simulink model "PD_controller_unit_test"  (R2018b)
settings: Solver=FixedStepAuto  StartTime=0.0  StopTime=100  FixedStep=simParams.sample_time_s  RelTol=1e-3
undefined symbols (not defined in the file): simParams
libraries: PD_Controller_Lib x1, control_command_generation_lib x1, satelliteDynamics_lib x1
settings Model: Creator=colem  LastModifiedBy=colem

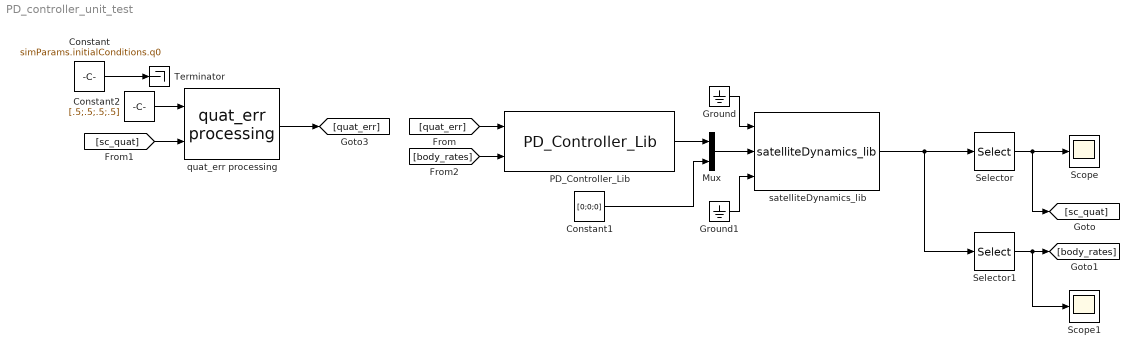
== system PD_controller_unit_test ==
  Constant : Constant  Value=simParams.initialConditions.q0
  Constant1 : Constant  Value=[0;0;0]
  Constant2 : Constant  Value=[.5;.5;.5;.5]
  Ground : Ground
  Ground1 : Ground
  Mux : Mux  Inputs=[3 3]
  PD_Controller_Lib : PD_Controller_Lib/PD_Controller_Lib  SystemSampleTime=-1
  Scope : Scope
  Scope1 : Scope
  Selector : Selector  InputPortWidth=13  IndexOptions=Index vector (dialog)  Indices=[7 8 9 10]  OutputSizes=1
  Selector1 : Selector  InputPortWidth=13  IndexOptions=Index vector (dialog)  Indices=[11 12 13]  OutputSizes=1
  Terminator : Terminator
  quat_err processing : control_command_generation_lib/control_command_generation_lib/quat_err processing  SystemSampleTime=-1
  satelliteDynamics_lib : satelliteDynamics_lib/satelliteDynamics_lib  SystemSampleTime=-1
  wires:
  quat_err processing/1 -> [quat_err]
  Constant/1 -> Terminator/1
  [sc_quat] -> quat_err processing/2
  [quat_err] -> PD_Controller_Lib/1
  satelliteDynamics_lib/1 -> Selector1/1, Selector/1
  Selector/1 -> [sc_quat], Scope/1
  Selector1/1 -> Scope1/1, [body_rates]
  [body_rates] -> PD_Controller_Lib/2
  Ground/1 -> satelliteDynamics_lib/1
  Ground1/1 -> satelliteDynamics_lib/3
  Constant1/1 -> Mux/2
  PD_Controller_Lib/1 -> Mux/1
  Mux/1 -> satelliteDynamics_lib/2
  Constant2/1 -> quat_err processing/1
